simulink library "LibDBC_Some_Node_ch0_ORIGINAL"  (Simulink 9.1)
settings: Solver=VariableStepAuto  StartTime=0.0  StopTime=10.0  RelTol=1e-3
undefined symbols (not defined in the file): bit_packing, bit_unpacking, IO_Blk_Lib_TTC500, IO_CAN_ConfigMsg
libraries: IOBlock_Library_TTC580 x4, simulink x2
(part 2 of 2)

== system LibDBC_Some_Node_ch0_ORIGINAL/Test_Message_integer/bit_packing1 ==
  Data_in : Inport
  bit_packing_s : S-Function  FunctionName=bit_packing_s  Parameters=SampleTime,Endianness,Format,Inversion,Startbit,Width_bits,Factor,Offset  SFunctionDeploymentMode=off  EnableBusSupport=off
  Data_out : Outport
  wires:
  Data_in/1 -> bit_packing_s/1
  bit_packing_s/1 -> Data_out/1

== system LibDBC_Some_Node_ch0_ORIGINAL/Test_Message_integer/bit_packing2 ==
  Data_in : Inport
  bit_packing_s : S-Function  FunctionName=bit_packing_s  Parameters=SampleTime,Endianness,Format,Inversion,Startbit,Width_bits,Factor,Offset  SFunctionDeploymentMode=off  EnableBusSupport=off
  Data_out : Outport
  wires:
  Data_in/1 -> bit_packing_s/1
  bit_packing_s/1 -> Data_out/1

== system LibDBC_Some_Node_ch0_ORIGINAL/Test_Message_integer/bit_packing3 ==
  Data_in : Inport
  bit_packing_s : S-Function  FunctionName=bit_packing_s  Parameters=SampleTime,Endianness,Format,Inversion,Startbit,Width_bits,Factor,Offset  SFunctionDeploymentMode=off  EnableBusSupport=off
  Data_out : Outport
  wires:
  Data_in/1 -> bit_packing_s/1
  bit_packing_s/1 -> Data_out/1

== system LibDBC_Some_Node_ch0_ORIGINAL/Test_Message_integer/bit_packing4 ==
  Data_in : Inport
  bit_packing_s : S-Function  FunctionName=bit_packing_s  Parameters=SampleTime,Endianness,Format,Inversion,Startbit,Width_bits,Factor,Offset  SFunctionDeploymentMode=off  EnableBusSupport=off
  Data_out : Outport
  wires:
  Data_in/1 -> bit_packing_s/1
  bit_packing_s/1 -> Data_out/1

== system LibDBC_Some_Node_ch0_ORIGINAL/Test_Message_integer/bit_packing5 ==
  Data_in : Inport
  bit_packing_s : S-Function  FunctionName=bit_packing_s  Parameters=SampleTime,Endianness,Format,Inversion,Startbit,Width_bits,Factor,Offset  SFunctionDeploymentMode=off  EnableBusSupport=off
  Data_out : Outport
  wires:
  Data_in/1 -> bit_packing_s/1
  bit_packing_s/1 -> Data_out/1
